simulink model "RobotX_FullSystemSep20"  (R2014a)
settings: Solver=FixedStepDiscrete  StartTime=0.0  StopTime=inf  FixedStep=.25  RelTol=1e-3
undefined symbols (not defined in the file): Com1, Com2, Com3, Com4, DiscIntNeverNeededParam, standard
libraries: simulink x11, xpcseriallib x11, slrtlib x3, speedgoatlib x1, speedgoatlib_IO102 x1
(part 3 of 4)

== system RobotX_FullSystemSep20/Main FSM/Acoustic FSM/Drive Pt3/Output Reassign ==
  "Valid " : Inport
  Data : Inport  Port=2
  Sensors : Inport  Port=3
  Acoustic Active : Constant
  Bus Creator2 : BusCreator  Inputs=3
  Bus Creator3 : BusCreator  Inputs=3
  Bus Creator5 : BusCreator  Inputs=2
  Constant3 : Constant
  Lidar Mode : Constant
  Outputs : Outport
  wires:
  Sensors/1 -> Bus Creator5/2  "Sensors"
  Bus Creator5/1 -> Outputs/1  "Output Signals"
  "Valid "/1 -> Bus Creator2/1  "Valid"
  Constant3/1 -> Bus Creator2/2  "Control Mode"
  Data/1 -> Bus Creator2/3  "Data"
  Bus Creator2/1 -> Bus Creator3/1  "Navigation Outputs"
  Acoustic Active/1 -> Bus Creator3/2  "Acoustic Active"
  Lidar Mode/1 -> Bus Creator3/3  "Lidar Mode"
  Bus Creator3/1 -> Bus Creator5/1  "Outputs"

== system RobotX_FullSystemSep20/Main FSM/Docking/Docking/Output Heirarchy ==
  Data : Inport
  Sensors : Inport  Port=2
  Acoustic Active : Constant  Value=0
  Bus Creator2 : BusCreator  Inputs=3
  Bus Creator3 : BusCreator  Inputs=3
  Bus Creator5 : BusCreator  Inputs=2
  Constant : Constant
  Constant3 : Constant
  Lidar Mode : Constant  Value=2
  Outputs : Outport
  wires:
  Sensors/1 -> Bus Creator5/2  "Sensors"
  Bus Creator5/1 -> Outputs/1  "Output Signals"
  Constant/1 -> Bus Creator2/1  "Valid"
  Constant3/1 -> Bus Creator2/2  "Control Mode"
  Data/1 -> Bus Creator2/3  "Data"
  Bus Creator2/1 -> Bus Creator3/1  "Navigation Outputs"
  Acoustic Active/1 -> Bus Creator3/2  "Acoustic Active"
  Lidar Mode/1 -> Bus Creator3/3  "Lidar Mode"
  Bus Creator3/1 -> Bus Creator5/1  "Outputs"

== system RobotX_FullSystemSep20/Main FSM/Docking/GPS Move/Output Reassign ==
  Vaild : Inport
  Data : Inport  Port=2
  Sensors : Inport  Port=3
  Acoustic Active : Constant  Value=0
  Bus Creator2 : BusCreator  Inputs=3
  Bus Creator3 : BusCreator  Inputs=3
  Bus Creator5 : BusCreator  Inputs=2
  Constant3 : Constant  Value=0
  Lidar Mode : Constant  Value=3
  Outputs : Outport
  wires:
  Sensors/1 -> Bus Creator5/2  "Sensors"
  Bus Creator5/1 -> Outputs/1  "Output Signals"
  Vaild/1 -> Bus Creator2/1  "Valid"
  Constant3/1 -> Bus Creator2/2  "Control Mode"
  Data/1 -> Bus Creator2/3  "Data"
  Bus Creator2/1 -> Bus Creator3/1  "Navigation Outputs"
  Acoustic Active/1 -> Bus Creator3/2  "Acoustic Active"
  Lidar Mode/1 -> Bus Creator3/3  "Lidar Mode"
  Bus Creator3/1 -> Bus Creator5/1  "Outputs"

== system RobotX_FullSystemSep20/Main FSM/Docking/Reverse/Output Heirarchy ==
  Sensors : Inport
  Acoustic Active : Constant  Value=0
  Bus Creator2 : BusCreator  Inputs=3
  Bus Creator3 : BusCreator  Inputs=3
  Bus Creator5 : BusCreator  Inputs=2
  Constant2 : Constant  Value=[-100; -100; 0; 0; 0; 0; 0; 0; 0; 0; 0; 0; 0; 0; 0; 0; 0; 0; 0; 0; 0; 0; 0; 0;]
  Constant3 : Constant
  Constant4 : Constant  Value=2
  Lidar Mode : Constant  Value=3
  Outputs : Outport
  wires:
  Sensors/1 -> Bus Creator5/2  "Sensors"
  Bus Creator5/1 -> Outputs/1  "Output Signals"
  Constant3/1 -> Bus Creator2/1  "Valid"
  Constant4/1 -> Bus Creator2/2  "Control Mode"
  Constant2/1 -> Bus Creator2/3  "Data"
  Bus Creator2/1 -> Bus Creator3/1  "Navigation Outputs"
  Acoustic Active/1 -> Bus Creator3/2  "Acoustic Active"
  Lidar Mode/1 -> Bus Creator3/3  "Lidar Mode"
  Bus Creator3/1 -> Bus Creator5/1  "Outputs"

== system RobotX_FullSystemSep20/Main FSM/Light Beacon/Approach/Output Reassign ==
  Vaild : Inport
  Data : Inport  Port=2
  Sensors : Inport  Port=3
  Acoustic Active : Constant  Value=0
  Bus Creator2 : BusCreator  Inputs=3
  Bus Creator3 : BusCreator  Inputs=3
  Bus Creator5 : BusCreator  Inputs=2
  Constant3 : Constant  Value=0
  Lidar Mode : Constant
  Outputs : Outport
  wires:
  Sensors/1 -> Bus Creator5/2  "Sensors"
  Bus Creator5/1 -> Outputs/1  "Output Signals"
  Vaild/1 -> Bus Creator2/1  "Valid"
  Constant3/1 -> Bus Creator2/2  "Control Mode"
  Data/1 -> Bus Creator2/3  "Data"
  Bus Creator2/1 -> Bus Creator3/1  "Navigation Outputs"
  Acoustic Active/1 -> Bus Creator3/2  "Acoustic Active"
  Lidar Mode/1 -> Bus Creator3/3  "Lidar Mode"
  Bus Creator3/1 -> Bus Creator5/1  "Outputs"

== system RobotX_FullSystemSep20/Main FSM/Light Beacon/GPS Move/Output Reassign ==
  Vaild : Inport
  Data : Inport  Port=2
  Sensors : Inport  Port=3
  Acoustic Active : Constant  Value=0
  Bus Creator2 : BusCreator  Inputs=3
  Bus Creator3 : BusCreator  Inputs=3
  Bus Creator5 : BusCreator  Inputs=2
  Constant3 : Constant  Value=0
  Lidar Mode : Constant
  Outputs : Outport
  wires:
  Sensors/1 -> Bus Creator5/2  "Sensors"
  Bus Creator5/1 -> Outputs/1  "Output Signals"
  Vaild/1 -> Bus Creator2/1  "Valid"
  Constant3/1 -> Bus Creator2/2  "Control Mode"
  Data/1 -> Bus Creator2/3  "Data"
  Bus Creator2/1 -> Bus Creator3/1  "Navigation Outputs"
  Acoustic Active/1 -> Bus Creator3/2  "Acoustic Active"
  Lidar Mode/1 -> Bus Creator3/3  "Lidar Mode"
  Bus Creator3/1 -> Bus Creator5/1  "Outputs"

== system RobotX_FullSystemSep20/Main FSM/Light Beacon/Spin	/Output Heirarchy ==
  Data : Inport
  Sensors : Inport  Port=2
  Acoustic Active : Constant  Value=0
  Bus Creator2 : BusCreator  Inputs=3
  Bus Creator3 : BusCreator  Inputs=3
  Bus Creator5 : BusCreator  Inputs=2
  Constant : Constant
  Constant3 : Constant
  Lidar Mode : Constant
  Outputs : Outport
  wires:
  Sensors/1 -> Bus Creator5/2  "Sensors"
  Bus Creator5/1 -> Outputs/1  "Output Signals"
  Constant/1 -> Bus Creator2/1  "Valid"
  Constant3/1 -> Bus Creator2/2  "Control Mode"
  Data/1 -> Bus Creator2/3  "Data"
  Bus Creator2/1 -> Bus Creator3/1  "Navigation Outputs"
  Acoustic Active/1 -> Bus Creator3/2  "Acoustic Active"
  Lidar Mode/1 -> Bus Creator3/3  "Lidar Mode"
  Bus Creator3/1 -> Bus Creator5/1  "Outputs"

== system RobotX_FullSystemSep20/Main FSM/Light Beacon/Stare/Output Heirarchy ==
  Data : Inport
  Lidar Mode : Inport  Port=2
  Sensors : Inport  Port=3
  Acoustic Active : Constant
  Bus Creator2 : BusCreator  Inputs=3
  Bus Creator3 : BusCreator  Inputs=3
  Bus Creator5 : BusCreator  Inputs=2
  Constant : Constant
  Constant3 : Constant
  Outputs : Outport
  wires:
  Sensors/1 -> Bus Creator5/2  "Sensors"
  Bus Creator5/1 -> Outputs/1  "Output Signals"
  Constant/1 -> Bus Creator2/1  "Valid"
  Constant3/1 -> Bus Creator2/2  "Control Mode"
  Data/1 -> Bus Creator2/3  "Data"
  Bus Creator2/1 -> Bus Creator3/1  "Navigation Outputs"
  Acoustic Active/1 -> Bus Creator3/2  "Acoustic Active"
  Lidar Mode/1 -> Bus Creator3/3  "Lidar Mode"
  Bus Creator3/1 -> Bus Creator5/1  "Outputs"

== system RobotX_FullSystemSep20/Main FSM/Start//Speedgate/GPS Move/Output Reassign ==
  Vaild : Inport
  Data : Inport  Port=2
  Sensors : Inport  Port=3
  Acoustic Active : Constant  Value=0
  Bus Creator2 : BusCreator  Inputs=3
  Bus Creator3 : BusCreator  Inputs=3
  Bus Creator5 : BusCreator  Inputs=2
  Constant3 : Constant  Value=0
  Lidar Mode : Constant
  Outputs : Outport
  wires:
  Sensors/1 -> Bus Creator5/2  "Sensors"
  Bus Creator5/1 -> Outputs/1  "Output Signals"
  Vaild/1 -> Bus Creator2/1  "Valid"
  Constant3/1 -> Bus Creator2/2  "Control Mode"
  Data/1 -> Bus Creator2/3  "Data"
  Bus Creator2/1 -> Bus Creator3/1  "Navigation Outputs"
  Acoustic Active/1 -> Bus Creator3/2  "Acoustic Active"
  Lidar Mode/1 -> Bus Creator3/3  "Lidar Mode"
  Bus Creator3/1 -> Bus Creator5/1  "Outputs"

== system RobotX_FullSystemSep20/Main FSM/Start//Speedgate/Speed Gate/Output Reassign ==
  Vaild : Inport
  Data : Inport  Port=2
  Sensors : Inport  Port=3
  Acoustic Active : Constant  Value=0
  Bus Creator2 : BusCreator  Inputs=3
  Bus Creator3 : BusCreator  Inputs=3
  Bus Creator5 : BusCreator  Inputs=2
  Constant3 : Constant  Value=0
  Lidar Mode : Constant
  Outputs : Outport
  wires:
  Sensors/1 -> Bus Creator5/2  "Sensors"
  Bus Creator5/1 -> Outputs/1  "Output Signals"
  Vaild/1 -> Bus Creator2/1  "Valid"
  Constant3/1 -> Bus Creator2/2  "Control Mode"
  Data/1 -> Bus Creator2/3  "Data"
  Bus Creator2/1 -> Bus Creator3/1  "Navigation Outputs"
  Acoustic Active/1 -> Bus Creator3/2  "Acoustic Active"
  Lidar Mode/1 -> Bus Creator3/3  "Lidar Mode"
  Bus Creator3/1 -> Bus Creator5/1  "Outputs"

== system RobotX_FullSystemSep20/Main FSM/Start//Speedgate/Start Gate/Output Reassign ==
  Vaild : Inport
  Data : Inport  Port=2
  Sensors : Inport  Port=3
  Acoustic Active : Constant  Value=0
  Bus Creator2 : BusCreator  Inputs=3
  Bus Creator3 : BusCreator  Inputs=3
  Bus Creator5 : BusCreator  Inputs=2
  Constant3 : Constant  Value=0
  Lidar Mode : Constant
  Outputs : Outport
  wires:
  Sensors/1 -> Bus Creator5/2  "Sensors"
  Bus Creator5/1 -> Outputs/1  "Output Signals"
  Vaild/1 -> Bus Creator2/1  "Valid"
  Constant3/1 -> Bus Creator2/2  "Control Mode"
  Data/1 -> Bus Creator2/3  "Data"
  Bus Creator2/1 -> Bus Creator3/1  "Navigation Outputs"
  Acoustic Active/1 -> Bus Creator3/2  "Acoustic Active"
  Lidar Mode/1 -> Bus Creator3/3  "Lidar Mode"
  Bus Creator3/1 -> Bus Creator5/1  "Outputs"

== matlab function RobotX_FullSystemSep20/Main FSM/Main Enabler ==
  data: taskSelector output; initEn output; startgateEn output; acousticEn output; dockingEn output; lightEn output; odoaEn output; termEn output; RCEn output; OnOffRCAuto input; mainTask input; initFin input; startgateFin input; acousticFin input; dockingFin input; lightFin input; odoaFin input
function [taskSelector,initEn,startgateEn,acousticEn,dockingEn,lightEn,...
    odoaEn,termEn,RCEn] = taskEnabler(OnOffRCAuto,mainTask,initFin,startgateFin,...
    acousticFin,dockingFin,lightFin,odoaFin)
%Written by Anderson Lebbad on July 19, 2013
%Last Edited: Edward Zhu on June 2, 2014
%   Substring search for task was written in
%   Case switches were redundant, combined with first set of if statements

%Changes the value of MainMode and the enablers for the tasks within the
%Main FSM.

% Currently cannot test light
lightFin = 1;
acousticFin = 1;
dockingFin = 1;
odoaFin = 1;

% Initialize enable signals
initEn = 0;
startgateEn = 0;
acousticEn = 0;
dockingEn = 0;
lightEn = 0;
odoaEn = 0;
termEn = 0;
RCEn = 0;

% Convert main task indicator to a string
mainTaskStr = char(mainTask);


% Adjust finished states based on user task selection (never skips
% initialization)
if ~isempty(strfind(mainTaskStr,'Acoustic'))
    startgateFin = 1;
elseif ~isempty(strfind(mainTaskStr,'Docking'))
    startgateFin = 1;
    acousticFin = 1;
elseif ~isempty(strfind(mainTaskStr,'Light'))
    startgateFin = 1;
    acousticFin = 1;
    dockingFin = 1;
elseif ~isempty(strfind(mainTaskStr,'ODOA'))
    startgateFin = 1;
    acousticFin = 1;
    dockingFin = 1;
    lightFin = 1;
end

% Set enable signals based on state completion
if initFin == 0
    initEn = 1;
    taskSelector = 1;
elseif OnOffRCAuto ~= 3
    RCEn = 1;
    taskSelector = 8;
elseif startgateFin == 0
    startgateEn = 1;
    taskSelector = 2;
elseif acousticFin == 0
    acousticEn = 1;
    taskSelector = 3;
elseif dockingFin == 0
    dockingEn = 1;
    taskSelector = 4;
elseif lightFin == 0
    lightEn = 1;
    taskSelector = 5;
elseif odoaFin == 0
    odoaEn = 1;
    taskSelector = 6;
else
    termEn = 1;
    taskSelector = 7;
end

end

== matlab function RobotX_FullSystemSep20/Main FSM/Docking/GPS Move/CalcTimes ==
  data: pts input; u input; Data output
function Data = calcTimes(pts, u)
%Written by Anderson Lebbad on August 9, 2014
%Last Edited: Dylan DeGaetano September 1, 2014

%Calculates times for the boat to get to points for a trajectory, and
%formats Data for communication

%Initialize
Data = zeros(24,1);
traj = zeros(8,3);
traj(:,1:2) = pts;



for k = 2:8
    %Calculate distance to travel from last point
    distTravel = sqrt(sum((pts(k-1,:)-pts(k,:)).^2));
    %Assume 1m per second speed
    traj(k,3) = traj(k-1,3) + distTravel;
    %Add time based off initial velocity to get to first point past initial
    if k == 2
        traj(k,3) = traj(k,3) + 2.5*abs(2-u);
    end
end


%Output Data
for i=1:8
    for j = 1:3
        Data(3*(i-1)+j) = traj(i,j);
    end
end

== matlab function RobotX_FullSystemSep20/Sensors/Serial In/Data Update ==
  data: Valid input; ControlMode input; V output; C output; Data input; D1 output; D2 output; D3 output; D4 output; D5 output; D6 output; D7 output; D8 output; D9 output; D10 output; D11 output; D12 output; D13 output; D14 output; D15 output; D16 output; D17 output; D18 output; D19 output; D20 output; D21 output; D22 output; D23 output; D24 output
function [V,C,D1,D2,D3,D4,D5,D6,D7,D8,D9,D10,D11,D12,D13,D14,D15,D16,D17,...
    D18,D19,D20,D21,D22,D23,D24] = dataSplit(Valid,ControlMode,Data)
%Written by Anderson Lebbad on August 10, 2014
%Last Edited by: Anderson Lebbad on September 11, 2014

%This function splits the data vector into the twelve channels it is
%composed of for communication

persistent HoldData

if isempty(HoldData)
    HoldData = zeros(26,1);
end

if Valid == 1
    HoldData(1) = Valid;
    HoldData(2) = ControlMode;
    HoldData(3) = Data(1);
    HoldData(4) = Data(2);
    HoldData(5) = Data(3);
    HoldData(6) = Data(4);
    HoldData(7) = Data(5);
    HoldData(8) = Data(6);
    HoldData(9) = Data(7);
    HoldData(10) = Data(8);
    HoldData(11) = Data(9);
    HoldData(12) = Data(10);
    HoldData(13) = Data(11);
    HoldData(14) = Data(12);
    HoldData(15) = Data(13);
    HoldData(16) = Data(14);
    HoldData(17) = Data(15);
    HoldData(18) = Data(16);
    HoldData(19) = Data(17);
    HoldData(20) = Data(18);
    HoldData(21) = Data(19);
    HoldData(22) = Data(20);
    HoldData(23) = Data(21);
    HoldData(24) = Data(22);
    HoldData(25) = Data(23);
    HoldData(26) = Data(24);
end

V = HoldData(1);
C = HoldData(2);
D1 = HoldData(3);
D2 = HoldData(4);
D3 = HoldData(5);
D4 = HoldData(6);
D5 = HoldData(7);
D6 = HoldData(8);
D7 = HoldData(9);
D8 = HoldData(10);
D9 = HoldData(11);
D10 = HoldData(12);
D11 = HoldData(13);
D12 = HoldData(14);
D13 = HoldData(15);
D14 = HoldData(16);
D15 = HoldData(17);
D16 = HoldData(18);
D17 = HoldData(19);
D18 = HoldData(20);
D19 = HoldData(21);
D20 = HoldData(22);
D21 = HoldData(23);
D22 = HoldData(24);
D23 = HoldData(25);
D24 = HoldData(26);

end

== matlab function RobotX_FullSystemSep20/Main FSM/Docking/GPS Move/GPSMove ==
  data: GoalNED input; X input; Finished output; valid output; Y input; Psi input; pts output
function [Finished,valid,pts] = GPSmove(GoalNED,X,Y,Psi)
%Written by Dylan DeGaetano on September 1, 2014
%Last edited by: Anderson Lebbad
%
%This function will go to a given NED cooridnate, last edit changed the
%goal pt and variable names

persistent Sample
if isempty(Sample)
Sample = 0;
end
Finished = 0;
pts = zeros(8,2);
%$Distance to object in meters

if Sample == 0
    pts(1,1) = X+5*cos(Psi*pi/180);
    pts(1,2) = Y+5*cos(Psi*pi/180);
    pts(8,1) = GoalNED(1,1);
    pts(8,2) = GoalNED(1,2);
    pts(2,:) = pts(1,:) +(1*(GoalNED-pts(1,:))/7);
    pts(3,:) = pts(1,:) +(2*(GoalNED-pts(1,:))/7);
    pts(4,:) = pts(1,:) +(3*(GoalNED-pts(1,:))/7);
    pts(5,:) = pts(1,:) +(4*(GoalNED-pts(1,:))/7);
    pts(6,:) = pts(1,:) +(5*(GoalNED-pts(1,:))/7);
    pts(7,:) = pts(1,:) +(6*(GoalNED-pts(1,:))/7);
    Sample = 1; 
    valid = 1;
    
else 
    range = sqrt(sum((GoalNED - [X Y]).^2));
    if range <= 5
        Finished = 1;
    end
    valid = 0;
end

== matlab function RobotX_FullSystemSep20/Main FSM/Docking/Dock Enabler ==
  data: taskSelector output; GpsEn output; DockEn output; ReverseEn output; mainTask input; GpsFin input; DockFin input
function [taskSelector,GpsEn,DockEn,ReverseEn]=Dock_Enabler(mainTask,GpsFin,DockFin)
%Written by Anderson Lebbad on July 19, 2013
%Last Edited: Dylan DeGaetano on September ,4 2014
%   Substring search for task was written in
%   Case switches were redundant, combined with first set of if statements

%Changes the value of MainMode and the enablers for the tasks within the
%Main FSM.

% Initialize enable signals
GpsEn = 0;
DockEn = 0;
ReverseEn = 0;

% Convert main task indicator to a string
mainTaskStr = char(mainTask);

% Adjust finished states based on user task selection (never skips
% initialization)
if ~isempty(strfind(mainTaskStr,'Dock'))
    GpsFin = 1;
elseif ~isempty(strfind(mainTaskStr,'reverse'))
    GpsFin = 1;
    DockFin = 1;
end

% Set enable signals based on state completion
if GpsFin == 0
    GpsEn = 1;
    taskSelector = 1;
elseif DockFin == 0
    DockEn = 1;
    taskSelector = 2;
else
    ReverseEn = 1 ;
    taskSelector = 3;
end

== matlab function RobotX_FullSystemSep20/Main FSM/Docking/Docking/MATLAB Function ==
  data: Finished output; X input; Data output; Y input; Psi input; Dist input; Angles input; idx input
function [Finished,Data] = Orient(X,Y,Psi,Dist,Angles,idx)
%Written by Dylan DeGaetano on September 2, 2014
%Last Edited By Anderson Lebbad on September 19 2014

%This function passes the current pose data with the requrested heading
%so that the boat is facing the Quay wall.This task must be in station
%keeping mode
%
%Anderson's edit moved the orient within this function and adjusts the code
%to work better with sensing information

persistent holdPose found

%Measured heading, from the target position to face the quay wall
QuayHeading = 97;

if isempty(holdPose)
    holdPose = [X Y QuayHeading];
    found = 0;
end

DistM=Dist(1)/100;
Finished = 0;

%Initialize Data variable
Data = zeros(24,1);

if found == 0
    if idx(1) ~= 0
        %Calculate the NED coordinate of the found symbol
        TargetX = X+DistM(idx(1))*cos((Psi+Angles(idx(1)))*pi/180);
        TargetY = Y+DistM(idx(1))*sin((Psi+Angles(idx(1)))*pi/180);
        %Set destination in front of dock to line up
        holdPose(1) = TargetX - 6*cos(QuayHeading*pi/180);
        holdPose(2) = TargetY - 6*sin(QuayHeading*pi/180);
        holdPose(3) = QuayHeading;
        %Track that the symbol has been found
        found = 1;
    end
else
    l1norm = abs(X-holdPose(1))+abs(Y-holdPose(2));
    if l1norm < 2
        %
        holdPose(1) = holdPose(1) + 6*cos(QuayHeading*pi/180);
        holdPose(2) = holdPose(2) + 6*sin(QuayHeading*pi/180);
        found = found + 1;
    end
end

if found >= 3
    holdPose = [X Y QuayHeading];
    Finished = 1;
end

Data(1) = holdPose(1);
Data(2) = holdPose(2);
Data(3) = holdPose(3);

== matlab function RobotX_FullSystemSep20/Main FSM/Acoustic FSM/Acoustics Pt1/Ping Point ==
  data: Deployed input; finished output; X input; Y input; Psi input; HorizBearing input; NewBearing input; Data output; acousticPose output
function [finished,Data,acousticPose] = PingPoint(Deployed,X,Y,Psi,HorizBearing,NewBearing)
%Written by Anderson Lebbad on September 12, 2014
%Last Edited:

%This function causes the vessel to spin in place until a ping is detected,
%then orients itself towards the direction of the source of that ping

persistent holdPose Pinged aveHeading aveXY

if isempty(holdPose)
    holdPose = [X Y Psi];
    Pinged = 0;
    aveHeading = [0 0]; %Two elements, first is running average, second is accumulator
    aveXY = [0 0]; %Two elements, X ave and Y ave
end

%Initialize output variables
finished = 0;
Data = zeros(24,1);


%Angular offset (indirect rate control)
offset = 5;

%Only move once flagged as deployed
if Deployed == 1
    %If it hasn't heard a ping yet, spin
    if Pinged == 0
        holdPose(3) = mod(Psi + offset,360);
    end
    
    %If the ping is less than 250 milliseconds (a timestep) then point at the
    %direction of sound
    if abs(HorizBearing) >= 15
        if NewBearing
            holdPose(3) = mod(Psi + HorizBearing,360);
            Pinged = 1;
        end
    end
    
    %If it gets a new acoustic sample, increment the running average
    if NewBearing
        aveHeading(2) = aveHeading(2) + 1;
        aveHeading(1) = (aveHeading(1)*(aveHeading(2)-1)+(Psi+HorizBearing))/aveHeading(2);
        %In case of drift, keep a running average of the XY coordinates as well
        aveXY(1) = (aveXY(1)*(aveHeading(2)-1)+X)/aveHeading(2);
        aveXY(2) = (aveXY(2)*(aveHeading(2)-1)+Y)/aveHeading(2);
    end
    
    if aveHeading(2) >= 16
        finished = 1;
    end
end

%Set desired pose
Data(1) = holdPose(1);
Data(2) = holdPose(2);
Data(3) = holdPose(3);

acousticPose = [aveXY aveHeading(1)];

== matlab function RobotX_FullSystemSep20/Main FSM/Start//Speedgate/Speed Gate/Calculate Times ==
  data: pts input; u input; Data output
function Data = calcTimes(pts, u)
%Written by Anderson Lebbad on August 9, 2014
%Last Edited:

%Calculates times for the boat to get to points for a trajectory, and
%formats Data for communication

%Initialize
Data = zeros(24,1);
traj = zeros(8,3);

pts8 = [pts(1,:); (pts(2,:)-pts(1,:))/3; 2*(pts(2,:)-pts(1,:))/3; pts(2,:);...
    (pts(3,:)-pts(2,:))/2; pts(3,:); (pts(4,:)-pts(3,:))/2; pts(4,:)];

traj(:,1:2) = pts8;

for k = 2:8
    %Calculate distance to travel from last point
    distTravel = sqrt(sum((pts8(k-1,:)-pts8(k,:)).^2));
    %Assume 1m per second speed
    traj(k,3) = traj(k-1,3) + distTravel;
    %Add time based off initial velocity to get to first point past initial
    if k == 2
        traj(k,3) = traj(k,3) + 2.5*abs(2-u);
    end
end


%Output Data
for i=1:8
    for j = 1:3
        Data(3*(i-1)+j) = traj(i,j);
    end
end

== matlab function RobotX_FullSystemSep20/Main FSM/Start//Speedgate/GPS Move/CalcTimes ==
  data: pts input; u input; Data output
function Data = calcTimes(pts, u)
%Written by Anderson Lebbad on August 9, 2014
%Last Edited: Dylan DeGaetano September 1, 2014

%Calculates times for the boat to get to points for a trajectory, and
%formats Data for communication

%Initialize
Data = zeros(24,1);
traj = zeros(8,3);
traj(:,1:2) = pts;



for k = 2:8
    %Calculate distance to travel from last point
    distTravel = sqrt(sum((pts(k-1,:)-pts(k,:)).^2));
    %Assume 1m per second speed
    traj(k,3) = traj(k-1,3) + distTravel;
    %Add time based off initial velocity to get to first point past initial
    if k == 2
        traj(k,3) = traj(k,3) + 2.5*abs(2-u);
    end
end


%Output Data
for i=1:8
    for j = 1:3
        Data(3*(i-1)+j) = traj(i,j);
    end
end

== matlab function RobotX_FullSystemSep20/Main FSM/Start//Speedgate/GPS Move/GPSMove ==
  data: GoalNED input; X input; Finished output; valid output; Y input; Psi input; pts output
function [Finished,valid,pts] = GPSmove(GoalNED,X,Y,Psi)
%Written by Dylan DeGaetano on September 1, 2014
%Last edited by: Anderson Lebbad
%
%This function will go to a given NED cooridnate, last edit changed the
%goal pt and variable names

persistent Sample
if isempty(Sample)
Sample = 0;
end
Finished = 0;
pts = zeros(8,2);
%$Distance to object in meters

if Sample == 0
    pts(1,1) = X+5*cos(Psi*pi/180);
    pts(1,2) = Y+5*cos(Psi*pi/180);
    pts(8,1) = GoalNED(1,1);
    pts(8,2) = GoalNED(1,2);
    pts(2,:) = pts(1,:) +(1*(GoalNED-pts(1,:))/7);
    pts(3,:) = pts(1,:) +(2*(GoalNED-pts(1,:))/7);
    pts(4,:) = pts(1,:) +(3*(GoalNED-pts(1,:))/7);
    pts(5,:) = pts(1,:) +(4*(GoalNED-pts(1,:))/7);
    pts(6,:) = pts(1,:) +(5*(GoalNED-pts(1,:))/7);
    pts(7,:) = pts(1,:) +(6*(GoalNED-pts(1,:))/7);
    Sample = 1; 
    valid = 1;
    
else 
    range = sqrt(sum((GoalNED - [X Y]).^2));
    if range <= 5
        Finished = 1;
    end
    valid = 0;
end

== matlab function RobotX_FullSystemSep20/Main FSM/Start//Speedgate/Main Enabler ==
  data: taskSelector output; GpsEn output; startEn output; speedEn output; ssgateTask input; GpsFin input; startFin input
function [taskSelector,GpsEn,startEn,speedEn]=Startgate_Enabler(ssgateTask,...
    GpsFin,startFin)
%Written by Anderson Lebbad on July 19, 2013
%Last Edited: Dylan DeGaetano on September ,4 2014
%   Substring search for task was written in
%   Case switches were redundant, combined with first set of if statements

%Changes the value of MainMode and the enablers for the tasks within the
%Main FSM.

% Initialize enable signals
GpsEn = 0;
startEn = 0;
speedEn = 0;

% Convert main task indicator to a string
ssgateTaskStr = char(ssgateTask);

% Adjust finished states based on user task selection (never skips
% initialization)
if ~isempty(strfind(ssgateTaskStr,'Start'))
    GpsFin = 1;
elseif ~isempty(strfind(ssgateTaskStr,'Speed'))
    GpsFin = 1;
    startFin = 1;
end

% Set enable signals based on state completion
if GpsFin == 0
    GpsEn = 1;
    taskSelector = 1;
elseif startFin == 0
    startEn = 1;
    taskSelector = 2;
else
    speedEn = 1 ;
    taskSelector = 3;
end

== matlab function RobotX_FullSystemSep20/Main FSM/Acoustic FSM/Acoustics Pt2/Ping Point ==
  data: Deployed input; finished output; X input; Y input; Psi input; HorizBearing input; NewBearing input; Data output; acousticPose output
function [finished,Data,acousticPose] = PingPoint(Deployed,X,Y,Psi,HorizBearing,NewBearing)
%Written by Anderson Lebbad on September 12, 2014
%Last Edited:

%This function causes the vessel to spin in place until a ping is detected,
%then orients itself towards the direction of the source of that ping

persistent holdPose Pinged aveHeading aveXY

if isempty(holdPose)
    holdPose = [X Y Psi];
    Pinged = 0;
    aveHeading = [0 0]; %Two elements, first is running average, second is accumulator
    aveXY = [0 0]; %Two elements, X ave and Y ave
end

%Initialize output variables
finished = 0;
Data = zeros(24,1);


%Angular offset (indirect rate control)
offset = 5;

%Only move once flagged as deployed
if Deployed == 1
    %If it hasn't heard a ping yet, spin
    if Pinged == 0
        holdPose(3) = mod(Psi + offset,360);
    end
    
    %If the ping is less than 250 milliseconds (a timestep) then point at the
    %direction of sound
    if abs(HorizBearing) >= 15
        if NewBearing
            holdPose(3) = mod(Psi + HorizBearing,360);
            Pinged = 1;
        end
    end
    
    %If it gets a new acoustic sample, increment the running average
    if NewBearing
        aveHeading(2) = aveHeading(2) + 1;
        aveHeading(1) = (aveHeading(1)*(aveHeading(2)-1)+(Psi+HorizBearing))/aveHeading(2);
        %In case of drift, keep a running average of the XY coordinates as well
        aveXY(1) = (aveXY(1)*(aveHeading(2)-1)+X)/aveHeading(2);
        aveXY(2) = (aveXY(2)*(aveHeading(2)-1)+Y)/aveHeading(2);
    end
    
    if aveHeading(2) >= 16
        finished = 1;
    end
end

%Set desired pose
Data(1) = holdPose(1);
Data(2) = holdPose(2);
Data(3) = holdPose(3);

acousticPose = [aveXY aveHeading(1)];

== matlab function RobotX_FullSystemSep20/Main FSM/Docking/GPS Move/LLA to NED ==
  data: GoalLLA input; GoalNED output; NED_origin input
function GoalNED = LLA2NED(GoalLLA,NED_origin)
%Written by Anderson Lebbad on September 20, 2014
%Last edited by:
%
%This function converts a target Latitude, Longitude, Altitude (LLA) point
%into North, East, Down (NED) coordinates

%First convert to earth centered, earth fixed frame
x_lla = [GoalLLA, 0]';
% LLE2ECEF: Converts from geodetic latitude, longitude, and altitude to earth-centered earth-fixed Cartesian coordinates
% INPUT: latitude phi (rad), longitude lambda (rad), altitude h (m)
% OUTPUT: [x, y, z]' (m) earth-centered earth-fixed Cartesian coordinates
a = 6378137; % equatorial radius of ellipsoid (semi-major axis) (m)
b = 6356752; % polar axis radius of ellipsoid (semi-minor axis) (m)

phi = x_lla(1);
lambda = x_lla(2);
h = x_lla(3);

% auxiliar quantities f, e, and N
f = (a-b)/a;
e = f*(2-f);
N = a/sqrt(1-(e*sin(phi))^2);
x_ecef = [(N+h)*cos(phi)*cos(lambda); (N+h)*cos(phi)*sin(lambda); (N*(1-e^2)+h)*sin(phi)];

% ECEF2NED Converts from earth-centered, earth-fixed Cartesian coordinates to tangent plane
% INPUT:
% 1) x_ecef=[x,y,z]' (m) earth-centered, earth-fixed Cartesian coordinates
% 2) ned_lla=[phi,lambda]' consiting of latitude phi (rad), longitude lambda (rad) of NED origin
% OUTPUT:
% 1) x_ned=[x,y,z]' (m) in NED coordinate system with the origin [phi,lambda]'

phi = NED_origin(1);
lambda = NED_origin(2);

% transformation  matrix
T = [-sin(phi)*cos(lambda) -sin(phi)*sin(lambda)  cos(phi)
    -sin(lambda)           cos(lambda)           0
    cos(phi)*cos(lambda)   cos(phi)*sin(lambda)  sin(phi)];
x_lla = [phi, lambda, 0]';
% LLE2ECEF: Converts from geodetic latitude, longitude, and altitude to earth-centered earth-fixed Cartesian coordinates
% INPUT: latitude phi (rad), longitude lambda (rad), altitude h (m)
% OUTPUT: [x, y, z]' (m) earth-centered earth-fixed Cartesian coordinates
a = 6378137; % equatorial radius of ellipsoid (semi-major axis) (m)
b = 6356752; % polar axis radius of ellipsoid (semi-minor axis) (m)

phi = x_lla(1);
lambda = x_lla(2);
h = x_lla(3);

% auxiliar quantities f, e, and N
f = (a-b)/a;
e = f*(2-f);
N = a/sqrt(1-(e*sin(phi))^2);
ecef_origin = [(N+h)*cos(phi)*cos(lambda); (N+h)*cos(phi)*sin(lambda); (N*(1-e^2)+h)*sin(phi)];

x_ned = T*(x_ecef-ecef_origin); % convert to NED
x_ned(3) = -x_ned(3);

GoalNED = x_ned(1:2)';

end

== matlab function RobotX_FullSystemSep20/Main FSM/Start//Speedgate/Speed Gate/Gate ==
  data: HeldHeading input; Finished output; Valid output; X input; Y input; Psi input; Dist input; Angles input; pts output; idx input
function [Finished, Valid, pts] = Gate(HeldHeading,X,Y,Psi,Dist,Angles,idx)
%Written by Anderson Lebbad on August 9, 2014
%Last Edited by:

%This function sends a forward trajectory (from the initial heading read
%into it) until a landmark is found. Once the landmark is found, a
%trajectory is written to dodge around it.

persistent Found finPt sample
if isempty(Found)
    Found = 0;
    finPt = [0 0];
    sample = 50;
end

dodgeLength = 15;
dodgeWidth = 5;
Finished = 0;
Valid = 0;
pts = zeros(4,2);
%Distance to object in meters
DistM = Dist/100;

%Set Valid bit. If it has been found in a previous timestep, the point is
%invalid, otherwise it is valid every increment of ts or if an object is
%found

%If no Landmark is found, navigate forward
if Found == 0
    %Initial pt
    pts(1,1) = X + 5*cos(HeldHeading*pi/180);
    pts(1,2) = Y + 5*sin(HeldHeading*pi/180);
    %Nothing found
    if idx(1) == 0
        pts(2,1) = X + 10*cos(HeldHeading*pi/180);
        pts(2,2) = Y + 10*sin(HeldHeading*pi/180);
        pts(3,1) = X + 15*cos(HeldHeading*pi/180);
        pts(3,2) = Y + 15*sin(HeldHeading*pi/180);
        pts(4,1) = X + 20*cos(HeldHeading*pi/180);
        pts(4,2) = Y + 20*sin(HeldHeading*pi/180);
        %Only flip valid bit every ts (seconds)
        sample = sample + 1;
        if sample >= 50
            Valid = 1;
            sample = 0;
        end
        %Something found
    elseif idx(2) == 0
        %Absolute Heading of object relative to boat's position
        landmarkHeading = mod((Psi + Angles(idx(1))),360);
        lmHeadingRad = landmarkHeading*pi/180;
        %Navigate to it
        pts(2,1) = X + DistM(idx(1))*cos(lmHeadingRad) - dodgeWidth*sin(lmHeadingRad);
        pts(2,2) = Y + DistM(idx(1))*sin(lmHeadingRad) + dodgeWidth*cos(lmHeadingRad);
        pts(3,1) = X + (DistM(idx(1)) + dodgeLength)*cos(lmHeadingRad);
        pts(3,2) = Y + (DistM(idx(1)) + dodgeLength)*sin(lmHeadingRad);
        pts(4,1) = X + (DistM(idx(1)) + 2*dodgeLength)*cos(lmHeadingRad);
        pts(4,2) = Y + (DistM(idx(1)) + 2*dodgeLength)*sin(lmHeadingRad);
        finPt = pts(4,:);
        %Flip valid if found
        Valid = 1;
        %Tag object as having been found
        Found = 1;
    else
        %Absolute Heading of object relative to boat's position
        landmarkHeading1 = mod((Psi + Angles(idx(1))),360);
        lmHeadingRad1 = landmarkHeading1*pi/180;
        landmarkHeading2 = mod((Psi + Angles(idx(2))),360);
        lmHeadingRad2 = landmarkHeading2*pi/180;
        %Landmark locations in NED
        lmX1 = X + DistM(idx(1))*cos(lmHeadingRad1);
        lmY1 = Y + DistM(idx(1))*sin(lmHeadingRad1);
        lmX2 = X + DistM(idx(2))*cos(lmHeadingRad2);
        lmY2 = Y + DistM(idx(2))*sin(lmHeadingRad2);
        %Middle point
        midX = (lmX1 + lmX2) / 2;
        midY = (lmY1 + lmY2) / 2;
        %Navigate to it
        pts(2,1) = midX;
        pts(2,2) = midY;
        %Hold heading and continue from midpoint
        pts(3,1) = midX + 5*cos(HeldHeading*pi/180);
        pts(3,2) = midY + 5*sin(HeldHeading*pi/180);
        pts(4,1) = midX + 10*cos(HeldHeading*pi/180);
        pts(4,2) = midY + 10*sin(HeldHeading*pi/180);
        finPt = pts(4,:);
        %Flip valid if found
        Valid = 1;
        %Tag object as having been found
        Found = 2;
    end
end

if Found == 1
    if idx(2) ~= 0
        %Absolute Heading of object relative to boat's position
        landmarkHeading1 = mod((Psi + Angles(idx(1))),360);
        lmHeadingRad1 = landmarkHeading1*pi/180;
        landmarkHeading2 = mod((Psi + Angles(idx(2))),360);
        lmHeadingRad2 = landmarkHeading2*pi/180;
        %Landmark locations in NED
        lmX1 = X + DistM(idx(1))*cos(lmHeadingRad1);
        lmY1 = Y + DistM(idx(1))*sin(lmHeadingRad1);
        lmX2 = X + DistM(idx(2))*cos(lmHeadingRad2);
        lmY2 = Y + DistM(idx(2))*sin(lmHeadingRad2);
        %Middle point
        midX = (lmX1 + lmX2) / 2;
        midY = (lmY1 + lmY2) / 2;
        %Navigate to it
        pts(2,1) = midX;
        pts(2,2) = midY;
        %Hold heading and continue from midpoint
        pts(3,1) = midX + 5*cos(HeldHeading*pi/180);
        pts(3,2) = midY + 5*sin(HeldHeading*pi/180);
        pts(4,1) = midX + 10*cos(HeldHeading*pi/180);
        pts(4,2) = midY + 10*sin(HeldHeading*pi/180);
        finPt = pts(4,:);
        %Flip valid if found
        Valid = 1;
        %Tag object as having been found
        Found = 2;
    end
end

%Check to see how far the current pose is from the final point in the
%trajectory
if Found >= 1
range = abs(finPt(1)-X)+abs(finPt(2)-Y);
else
    range = 1000;
end
if range <= 5
    Finished = 1;
end

end

== matlab function RobotX_FullSystemSep20/Main FSM/Start//Speedgate/GPS Move/LLA to NED ==
  data: GoalLLA input; GoalNED output; NED_origin input
function GoalNED = LLA2NED(GoalLLA,NED_origin)
%Written by Anderson Lebbad on September 20, 2014
%Last edited by:
%
%This function converts a target Latitude, Longitude, Altitude (LLA) point
%into North, East, Down (NED) coordinates

%First convert to earth centered, earth fixed frame
x_lla = [GoalLLA, 0]';
% LLE2ECEF: Converts from geodetic latitude, longitude, and altitude to earth-centered earth-fixed Cartesian coordinates
% INPUT: latitude phi (rad), longitude lambda (rad), altitude h (m)
% OUTPUT: [x, y, z]' (m) earth-centered earth-fixed Cartesian coordinates
a = 6378137; % equatorial radius of ellipsoid (semi-major axis) (m)
b = 6356752; % polar axis radius of ellipsoid (semi-minor axis) (m)

phi = x_lla(1);
lambda = x_lla(2);
h = x_lla(3);

% auxiliar quantities f, e, and N
f = (a-b)/a;
e = f*(2-f);
N = a/sqrt(1-(e*sin(phi))^2);
x_ecef = [(N+h)*cos(phi)*cos(lambda); (N+h)*cos(phi)*sin(lambda); (N*(1-e^2)+h)*sin(phi)];

% ECEF2NED Converts from earth-centered, earth-fixed Cartesian coordinates to tangent plane
% INPUT:
% 1) x_ecef=[x,y,z]' (m) earth-centered, earth-fixed Cartesian coordinates
% 2) ned_lla=[phi,lambda]' consiting of latitude phi (rad), longitude lambda (rad) of NED origin
% OUTPUT:
% 1) x_ned=[x,y,z]' (m) in NED coordinate system with the origin [phi,lambda]'

phi = NED_origin(1);
lambda = NED_origin(2);

% transformation  matrix
T = [-sin(phi)*cos(lambda) -sin(phi)*sin(lambda)  cos(phi)
    -sin(lambda)           cos(lambda)           0
    cos(phi)*cos(lambda)   cos(phi)*sin(lambda)  sin(phi)];
x_lla = [phi, lambda, 0]';
% LLE2ECEF: Converts from geodetic latitude, longitude, and altitude to earth-centered earth-fixed Cartesian coordinates
% INPUT: latitude phi (rad), longitude lambda (rad), altitude h (m)
% OUTPUT: [x, y, z]' (m) earth-centered earth-fixed Cartesian coordinates
a = 6378137; % equatorial radius of ellipsoid (semi-major axis) (m)
b = 6356752; % polar axis radius of ellipsoid (semi-minor axis) (m)

phi = x_lla(1);
lambda = x_lla(2);
h = x_lla(3);

% auxiliar quantities f, e, and N
f = (a-b)/a;
e = f*(2-f);
N = a/sqrt(1-(e*sin(phi))^2);
ecef_origin = [(N+h)*cos(phi)*cos(lambda); (N+h)*cos(phi)*sin(lambda); (N*(1-e^2)+h)*sin(phi)];

x_ned = T*(x_ecef-ecef_origin); % convert to NED
x_ned(3) = -x_ned(3);

GoalNED = x_ned(1:2)';

end

== matlab function RobotX_FullSystemSep20/Main FSM/Acoustic FSM/Acoustics Pt3/Ping Point ==
  data: Deployed input; finished output; X input; Y input; Psi input; HorizBearing input; NewBearing input; Data output; acousticPose output
function [finished,Data,acousticPose] = PingPoint(Deployed,X,Y,Psi,HorizBearing,NewBearing)
%Written by Anderson Lebbad on September 12, 2014
%Last Edited:

%This function causes the vessel to spin in place until a ping is detected,
%then orients itself towards the direction of the source of that ping

persistent holdPose Pinged aveHeading aveXY

if isempty(holdPose)
    holdPose = [X Y Psi];
    Pinged = 0;
    aveHeading = [0 0]; %Two elements, first is running average, second is accumulator
    aveXY = [0 0]; %Two elements, X ave and Y ave
end

%Initialize output variables
finished = 0;
Data = zeros(24,1);


%Angular offset (indirect rate control)
offset = 5;

%Only move once flagged as deployed
if Deployed == 1
    %If it hasn't heard a ping yet, spin
    if Pinged == 0
        holdPose(3) = mod(Psi + offset,360);
    end
    
    %If the ping is less than 250 milliseconds (a timestep) then point at the
    %direction of sound
    if abs(HorizBearing) >= 15
        if NewBearing
            holdPose(3) = mod(Psi + HorizBearing,360);
            Pinged = 1;
        end
    end
    
    %If it gets a new acoustic sample, increment the running average
    if NewBearing
        aveHeading(2) = aveHeading(2) + 1;
        aveHeading(1) = (aveHeading(1)*(aveHeading(2)-1)+(Psi+HorizBearing))/aveHeading(2);
        %In case of drift, keep a running average of the XY coordinates as well
        aveXY(1) = (aveXY(1)*(aveHeading(2)-1)+X)/aveHeading(2);
        aveXY(2) = (aveXY(2)*(aveHeading(2)-1)+Y)/aveHeading(2);
    end
    
    if aveHeading(2) >= 16
        finished = 1;
    end
end

%Set desired pose
Data(1) = holdPose(1);
Data(2) = holdPose(2);
Data(3) = holdPose(3);

acousticPose = [aveXY aveHeading(1)];

== matlab function RobotX_FullSystemSep20/Main FSM/Light Beacon/Approach/Approach ==
  data: X input; Finished output; valid output; Y input; Psi input; Dist input; pts output; Angles input; idx input
function [Finished,valid,pts] = Approach(X,Y,Psi,Dist,Angles,idx)
%Written by Dylan DeGaetano on September 1, 2014
%Last edited by: Dylan DeGaetano on September 10, 2014
%
%This function will move to the light Buoy, current it will switch once it
%is 7m away to the stare function.

persistent Sample GoalPts

if isempty(Sample)
    Sample = 0;
    GoalPts =zeros(1,2);
end

Finished = 0;
pts = zeros(8,2);
valid = 0;

%$Distance to object in meters
DistM = Dist/100;

if Sample == 0
    if idx(1) ~= 0
        targetHeading = (Psi + Angles(idx(1)))*pi/180;
        TargetX = X + (DistM(idx(1))-8) * cos(targetHeading);
        TargetY = Y + (DistM(idx(1))-8) * sin(targetHeading);
        GoalPts(1,1) = TargetX;
        GoalPts(1,2) = TargetY;
        pts(1,1) = X + 5 * cos(Psi * pi/180);
        pts(1,2) = Y + 5 * cos(Psi * pi/180);
        pts(8,1) = GoalPts(1,1);
        pts(8,2) = GoalPts(1,2);
        pts(2,:) = pts(1,:) + (1 * (GoalPts - pts(1,:))/7);
        pts(3,:) = pts(1,:) + (2 * (GoalPts - pts(1,:))/7);
        pts(4,:) = pts(1,:) + (3 * (GoalPts - pts(1,:))/7);
        pts(5,:) = pts(1,:) + (4 * (GoalPts - pts(1,:))/7);
        pts(6,:) = pts(1,:) + (5 * (GoalPts - pts(1,:))/7);
        pts(7,:) = pts(1,:) + (6 * (GoalPts - pts(1,:))/7);
        Sample = 1;
        valid = 1;
    end
    
else
    range = sqrt(sum((GoalPts - [X Y]).^2));
    if range <= 7
        Finished = 1;
    end
    valid=1;
end

== matlab function RobotX_FullSystemSep20/Main FSM/Acoustic FSM/Drive Pt2/CalcTimes ==
  data: pts input; u input; Data output
function Data = calcTimes(pts, u)
%Written by Anderson Lebbad on August 9, 2014
%Last Edited: Dylan DeGaetano September 1, 2014

%Calculates times for the boat to get to points for a trajectory, and
%formats Data for communication

%Initialize
Data = zeros(24,1);
traj = zeros(8,3);
traj(:,1:2) = pts;



for k = 2:8
    %Calculate distance to travel from last point
    distTravel = sqrt(sum((pts(k-1,:)-pts(k,:)).^2));
    %Assume 1m per second speed
    traj(k,3) = traj(k-1,3) + distTravel;
    %Add time based off initial velocity to get to first point past initial
    if k == 2
        traj(k,3) = traj(k,3) + 2.5*abs(2-u);
    end
end


%Output Data
for i=1:8
    for j = 1:3
        Data(3*(i-1)+j) = traj(i,j);
    end
end

== matlab function RobotX_FullSystemSep20/Main FSM/Acoustic FSM/Drive Pt2/GPSMove ==
  data: X input; Finished output; valid output; Y input; Psi input; GoalPt input; pts output
function [Finished, valid, pts] = GPSmove(X,Y,Psi,GoalPt)
%Written by Dylan DeGaetano on September 1, 2014
%Last edited by: Michael Benson on September 4, 2014
%   Changed Sample to be a persistent variable so that pts will not be
%   recalculated every iteration.
%
%This function will go to a given NED cooridnate 



persistent Sample

if isempty(Sample)
    Sample = 0;
end

valid = 0;
Finished = 0;
pts = zeros(8,2);
%$Distance to object in meters

if Sample == 0
    valid = 1;
    pts(1,1) = X+5*cos(Psi*pi/180);
    pts(1,2) = Y+5*cos(Psi*pi/180);
    pts(8,1) = GoalPt(1,1);
    pts(8,2) = GoalPt(1,2);
    pts(2,:) = pts(1,:) +(1*(GoalPt-pts(1,:))/7);
    pts(3,:) = pts(1,:) +(2*(GoalPt-pts(1,:))/7);
    pts(4,:) = pts(1,:) +(3*(GoalPt-pts(1,:))/7);
    pts(5,:) = pts(1,:) +(4*(GoalPt-pts(1,:))/7);
    pts(6,:) = pts(1,:) +(5*(GoalPt-pts(1,:))/7);
    pts(7,:) = pts(1,:) +(6*(GoalPt-pts(1,:))/7);
    Sample = 1; 
else 
    range = sqrt(sum((GoalPt - [X Y]).^2));
    if range <= 3
        Finished = 1;
    end
end

== matlab function RobotX_FullSystemSep20/Main FSM/Light Beacon/Spin	/Spin ==
  data: Finished output; time input; X input; Data output; Y input; Psi input; Angles input; Found output; idx input
function [Finished, Data, Found] = Spin(time, X, Y, Psi, Angles, idx)
%Written by Anderson Lebbad on August 9, 2014
%Last Edited:Dylan DeGaetano on September 8, 2014

%This function passes the current pose data with a heading offset as the
%desired pose for the station keeping controller to use. if the Lidar finds
%the bouy a found singal will be set high. 

persistent holdPose startHeading

if isempty(holdPose) && isempty(startHeading)
    holdPose = [X Y Psi];
    startHeading = Psi;   
end

Found = 0;

if time > 10 && abs(Psi - startHeading) < 5
    Finished = 1;
else
    Finished = 0;
end

%Initialize Data variable
Data = zeros(24,1);

if idx(1) == 0 %if nothing has been found
    %Angular offset (indirect rate control)
    offset = 30;
    
    holdPose(3) = mod(Psi + offset,360);
    
    %Set desired pose
    Data(1,1) = holdPose(1);
    Data(2,1) = holdPose(2);
    Data(3,1) = holdPose(3);
       
else %we found the bouy
    Data(1,1) = holdPose(1);
    Data(2,1) = holdPose(2);
    Data(3,1) = Psi+Angles(idx(1));
    Found = 1;
end

== matlab function RobotX_FullSystemSep20/Main FSM/Light Beacon/GPS Move/LLA to NED1 ==
  data: GoalLLA input; GoalNED output; NED_origin input
function GoalNED = LLA2NED(GoalLLA,NED_origin)
%Written by Anderson Lebbad on September 20, 2014
%Last edited by:
%
%This function converts a target Latitude, Longitude, Altitude (LLA) point
%into North, East, Down (NED) coordinates

%First convert to earth centered, earth fixed frame
x_lla = [GoalLLA, 0]';
% LLE2ECEF: Converts from geodetic latitude, longitude, and altitude to earth-centered earth-fixed Cartesian coordinates
% INPUT: latitude phi (rad), longitude lambda (rad), altitude h (m)
% OUTPUT: [x, y, z]' (m) earth-centered earth-fixed Cartesian coordinates
a = 6378137; % equatorial radius of ellipsoid (semi-major axis) (m)
b = 6356752; % polar axis radius of ellipsoid (semi-minor axis) (m)

phi = x_lla(1);
lambda = x_lla(2);
h = x_lla(3);

% auxiliar quantities f, e, and N
f = (a-b)/a;
e = f*(2-f);
N = a/sqrt(1-(e*sin(phi))^2);
x_ecef = [(N+h)*cos(phi)*cos(lambda); (N+h)*cos(phi)*sin(lambda); (N*(1-e^2)+h)*sin(phi)];

% ECEF2NED Converts from earth-centered, earth-fixed Cartesian coordinates to tangent plane
% INPUT:
% 1) x_ecef=[x,y,z]' (m) earth-centered, earth-fixed Cartesian coordinates
% 2) ned_lla=[phi,lambda]' consiting of latitude phi (rad), longitude lambda (rad) of NED origin
% OUTPUT:
% 1) x_ned=[x,y,z]' (m) in NED coordinate system with the origin [phi,lambda]'

phi = ned_lla(1);
lambda = ned_lla(2);

% transformation  matrix
T = [-sin(phi)*cos(lambda) -sin(phi)*sin(lambda)  cos(phi)
    -sin(lambda)           cos(lambda)           0
    cos(phi)*cos(lambda)   cos(phi)*sin(lambda)  sin(phi)];
x_lla = [phi, lambda, 0]';
% LLE2ECEF: Converts from geodetic latitude, longitude, and altitude to earth-centered earth-fixed Cartesian coordinates
% INPUT: latitude phi (rad), longitude lambda (rad), altitude h (m)
% OUTPUT: [x, y, z]' (m) earth-centered earth-fixed Cartesian coordinates
a = 6378137; % equatorial radius of ellipsoid (semi-major axis) (m)
b = 6356752; % polar axis radius of ellipsoid (semi-minor axis) (m)

phi = x_lla(1);
lambda = x_lla(2);
h = x_lla(3);

% auxiliar quantities f, e, and N
f = (a-b)/a;
e = f*(2-f);
N = a/sqrt(1-(e*sin(phi))^2);
ecef_origin = [(N+h)*cos(phi)*cos(lambda); (N+h)*cos(phi)*sin(lambda); (N*(1-e^2)+h)*sin(phi)];

x_ned = T*(x_ecef-ecef_origin); % convert to NED
x_ned(3) = -x_ned(3);

GoalNED = x_ned(1:2)';

end

== matlab function RobotX_FullSystemSep20/Main FSM/Acoustic FSM/Drive Pt3/CalcTimes ==
  data: pts input; u input; Data output
function Data = calcTimes(pts, u)
%Written by Anderson Lebbad on August 9, 2014
%Last Edited: Dylan DeGaetano September 1, 2014

%Calculates times for the boat to get to points for a trajectory, and
%formats Data for communication

%Initialize
Data = zeros(24,1);
traj = zeros(8,3);
traj(:,1:2) = pts;



for k = 2:8
    %Calculate distance to travel from last point
    distTravel = sqrt(sum((pts(k-1,:)-pts(k,:)).^2));
    %Assume 1m per second speed
    traj(k,3) = traj(k-1,3) + distTravel;
    %Add time based off initial velocity to get to first point past initial
    if k == 2
        traj(k,3) = traj(k,3) + 2.5*abs(2-u);
    end
end


%Output Data
for i=1:8
    for j = 1:3
        Data(3*(i-1)+j) = traj(i,j);
    end
end

== matlab function RobotX_FullSystemSep20/Main FSM/Acoustic FSM/Drive Pt3/GPSMove ==
  data: X input; Finished output; valid output; Y input; Psi input; GoalPt input; pts output
function [Finished, valid, pts] = GPSmove(X,Y,Psi,GoalPt)
%Written by Dylan DeGaetano on September 1, 2014
%Last edited by: Michael Benson on September 4, 2014
%   Changed Sample to be a persistent variable so that pts will not be
%   recalculated every iteration.
%
%This function will go to a given NED cooridnate 



persistent Sample

if isempty(Sample)
    Sample = 0;
end

valid = 0;
Finished = 0;
pts = zeros(8,2);
%$Distance to object in meters

if Sample == 0
    valid = 1;
    pts(1,1) = X+5*cos(Psi*pi/180);
    pts(1,2) = Y+5*cos(Psi*pi/180);
    pts(8,1) = GoalPt(1,1);
    pts(8,2) = GoalPt(1,2);
    pts(2,:) = pts(1,:) +(1*(GoalPt-pts(1,:))/7);
    pts(3,:) = pts(1,:) +(2*(GoalPt-pts(1,:))/7);
    pts(4,:) = pts(1,:) +(3*(GoalPt-pts(1,:))/7);
    pts(5,:) = pts(1,:) +(4*(GoalPt-pts(1,:))/7);
    pts(6,:) = pts(1,:) +(5*(GoalPt-pts(1,:))/7);
    pts(7,:) = pts(1,:) +(6*(GoalPt-pts(1,:))/7);
    Sample = 1; 
else 
    range = sqrt(sum((GoalPt - [X Y]).^2));
    if range <= 3
        Finished = 1;
    end
end

== matlab function RobotX_FullSystemSep20/Main FSM/Acoustic FSM/Point/Point ==
  data: AcousticPose1 input; AcousticPose2 input; AcousticPose3 input; PingPose output
function PingPose  = PingPoint(AcousticPose1,AcousticPose2,AcousticPose3)
%Written by Anderson Lebbad on September 13, 2014
%Last Edited:

%This function causes the vessel point at the estimated location of the
%pinger

%% Calculate the NED point by finding the three intersections and averaging

%First intersection
compMat = [cos(AcousticPose1(3)), sin(AcousticPose1(3)); cos(AcousticPose2(3)), sin(AcousticPose2(3))];
intScales = [(AcousticPose2(1)-AcousticPose1(1)), (AcousticPose2(2)-AcousticPose1(2))]/compMat;
pingPose1 = [(AcousticPose1(1)+intScales(1)*compMat(1,1)), (AcousticPose1(2)+intScales(1)*compMat(1,2))];

%Second intersection
compMat = [cos(AcousticPose1(3)), sin(AcousticPose1(3)); cos(AcousticPose3(3)), sin(AcousticPose3(3))];
intScales = [(AcousticPose3(1)-AcousticPose1(1)), (AcousticPose3(2)-AcousticPose1(2))]/compMat;
pingPose2 = [(AcousticPose1(1)+intScales(1)*compMat(1,1)), (AcousticPose1(2)+intScales(1)*compMat(1,2))];

%Second intersection
compMat = [cos(AcousticPose2(3)) sin(AcousticPose2(3)); cos(AcousticPose3(3)) sin(AcousticPose3(3))];
intScales = [(AcousticPose3(1)-AcousticPose2(1)), (AcousticPose3(2)-AcousticPose2(2))]/compMat;
pingPose3 = [(AcousticPose2(1)+intScales(1)*compMat(1,1)), (AcousticPose2(2)+intScales(1)*compMat(1,2))];

PingPose = (pingPose1+pingPose2+pingPose3)/3;

end
